simulink model "test"  (R2020a)
settings: Solver=FixedStepDiscrete  StartTime=0.0  StopTime=10.0  RelTol=1e-3
settings Model: Creator=김진성  LastModifiedBy=김진성
settings OptimizationCC: EnhancedBackFolding=on  PassReuseOutputArgsAs=Individual arguments  OptimizeBlockOrder=speed  DifferentSizesBufferReuse=on  OptimizationCustomize=off  EfficientTunableParamExpr=on
settings DebuggingCC: ParameterTunabilityLossMsg=error
settings HardwareCC: ProdBitPerPointer=32  ProdBitPerSizeT=32  ProdBitPerPtrDiffT=32  ProdLargestAtomicInteger=Long  ProdLargestAtomicFloat=Double  ProdWordSize=32  ProdHWDeviceType=ARM Compatible->ARM Cortex
settings SFSimCC: MATLABDynamicMemAlloc=off
settings RTWCC: SystemTargetFile=ert.tlc  GenCodeOnly=on  TemplateMakefile=ert_default_tmf  GenerateReport=on  IncludeHyperlinkInReport=on  LaunchReport=on  GenerateTraceInfo=on  GenerateTraceReport=on  GenerateTraceReportSl=on  GenerateTraceReportSf=on  GenerateTraceReportEml=on  GenerateCodeMetricsReport=on  GenerateCodeReplacementReport=on
settings CodeAppCC: ForceParamTrailComments=on  IgnoreCustomStorageClasses=off  OperatorAnnotations=on  SimulinkDataObjDesc=on  SFDataObjDesc=on  InsertBlockDesc=on
settings ERTTargetCC: TargetLangStandard=C99 (ISO)  GenerateSampleERTMain=on  MultiInstanceERTCode=on  CodeInterfacePackaging=Reusable function  ERTCustomFileTemplate=example_file_process.tlc

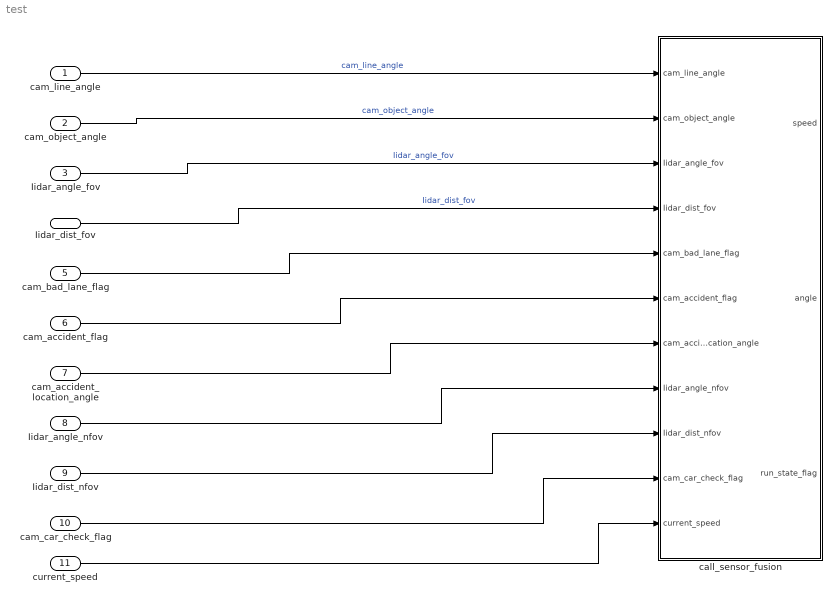
== system test ==
  cam_line_angle : Inport
  cam_object_angle : Inport  Port=2
  Iidar_angle_fov : Inport  Port=3
  Iidar_dist_fov : Inport  Port=4
  cam_bad_lane_flag : Inport  Port=5
  cam_accident_flag : Inport  Port=6
  cam_accident_location_angle : Inport  Port=7
  Iidar_angle_nfov : Inport  Port=8
  Iidar_dist_nfov : Inport  Port=9
  cam_car_check_flag : Inport  Port=10
  current_speed : Inport  Port=11
  call_sensor_fusion : Subsystem  TreatAsAtomicUnit=on
      settings: RTWSystemCode=Nonreusable function  RTWFcnNameOpts=Use subsystem name
  wires:
  cam_accident_location_angle/1 -> call_sensor_fusion/7(cam_accident_location_angle)
  cam_line_angle/1 -> call_sensor_fusion/1(cam_line_angle)  "cam_line_angle"
  cam_object_angle/1 -> call_sensor_fusion/2(cam_object_angle)  "cam_object_angle"
  Iidar_angle_fov/1 -> call_sensor_fusion/3(Iidar_angle_fov)  "Iidar_angle_fov"
  Iidar_dist_fov/1 -> call_sensor_fusion/4(Iidar_dist_fov)  "Iidar_dist_fov"
  Iidar_angle_nfov/1 -> call_sensor_fusion/8(Iidar_angle_nfov)
  Iidar_dist_nfov/1 -> call_sensor_fusion/9(Iidar_dist_nfov)
  cam_bad_lane_flag/1 -> call_sensor_fusion/5(cam_bad_lane_flag)
  cam_accident_flag/1 -> call_sensor_fusion/6(cam_accident_flag)
  cam_car_check_flag/1 -> call_sensor_fusion/10(cam_car_check_flag)
  current_speed/1 -> call_sensor_fusion/11(current_speed)

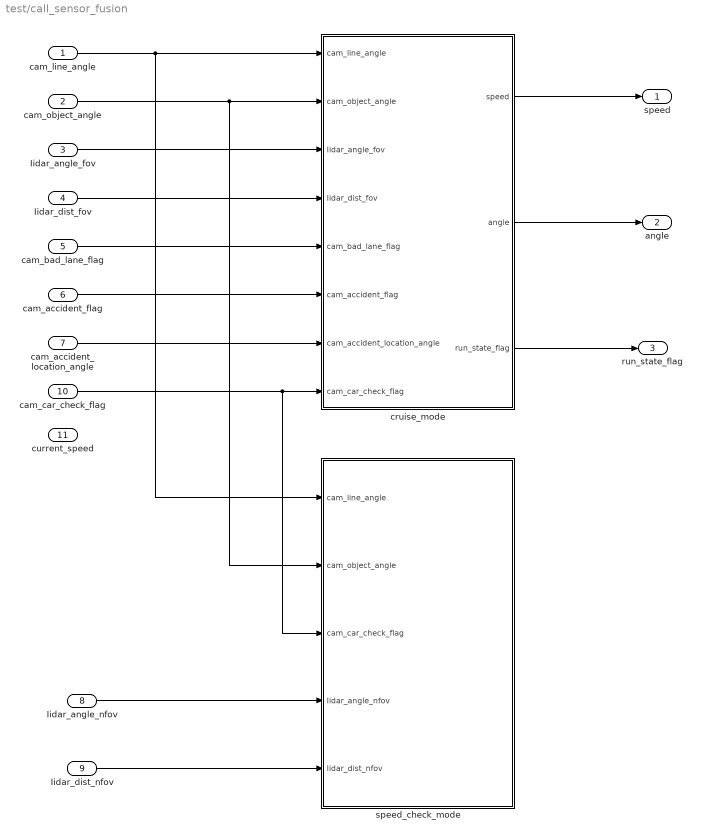
== system test/call_sensor_fusion ==
  cam_line_angle : Inport
  cam_object_angle : Inport  Port=2
  Iidar_angle_fov : Inport  Port=3
  Iidar_dist_fov : Inport  Port=4
  cam_bad_lane_flag : Inport  Port=5
  cam_accident_flag : Inport  Port=6
  cam_accident_location_angle : Inport  Port=7
  Iidar_angle_nfov : Inport  Port=8
  Iidar_dist_nfov : Inport  Port=9
  cam_car_check_flag : Inport  Port=10
  current_speed : Inport  Port=11
  cruise_mode : Subsystem  TreatAsAtomicUnit=on
      settings: RTWFcnNameOpts=Use subsystem name
  speed_check_mode : Subsystem
  speed : Outport
  angle : Outport  Port=2
  run_state_flag : Outport  Port=3
  wires:
  Iidar_angle_fov/1 -> cruise_mode/3(Iidar_angle_fov)
  Iidar_dist_fov/1 -> cruise_mode/4(Iidar_dist_fov)
  Iidar_angle_nfov/1 -> speed_check_mode/4(Iidar_angle_nfov)
  Iidar_dist_nfov/1 -> speed_check_mode/5(Iidar_dist_nfov)
  cruise_mode/2(angle) -> angle/1
  cruise_mode/1(speed) -> speed/1
  cruise_mode/3(run_state_flag) -> run_state_flag/1
  cam_line_angle/1 -> speed_check_mode/1(cam_line_angle), cruise_mode/1(cam_line_angle)
  cam_object_angle/1 -> speed_check_mode/2(cam_object_angle), cruise_mode/2(cam_object_angle)
  cam_bad_lane_flag/1 -> cruise_mode/5(cam_bad_lane_flag)
  cam_accident_flag/1 -> cruise_mode/6(cam_accident_flag)
  cam_accident_location_angle/1 -> cruise_mode/7(cam_accident_location_angle)
  cam_car_check_flag/1 -> speed_check_mode/3(cam_car_check_flag), cruise_mode/8(cam_car_check_flag)

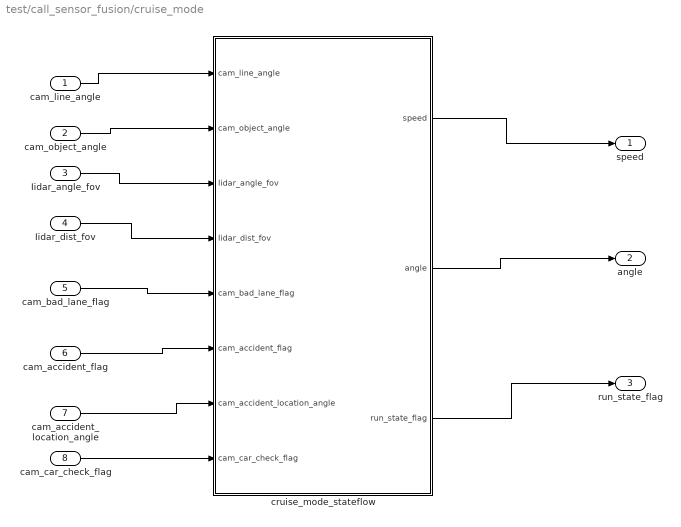
== system test/call_sensor_fusion/cruise_mode ==
  cam_line_angle : Inport
  cam_object_angle : Inport  Port=2
  Iidar_angle_fov : Inport  Port=3
  Iidar_dist_fov : Inport  Port=4
  cam_bad_lane_flag : Inport  Port=5
  cam_accident_flag : Inport  Port=6
  cam_accident_location_angle : Inport  Port=7
  cam_car_check_flag : Inport  Port=8
  cruise_mode_stateflow : Stateflow chart  TreatAsAtomicUnit=on
      settings: RTWSystemCode=Nonreusable function  RTWFcnNameOpts=Use subsystem name
  speed : Outport
  angle : Outport  Port=2
  run_state_flag : Outport  Port=3
  wires:
  cam_line_angle/1 -> cruise_mode_stateflow/1(cam_line_angle)
  cam_object_angle/1 -> cruise_mode_stateflow/2(cam_object_angle)
  cruise_mode_stateflow/1(speed) -> speed/1
  cruise_mode_stateflow/2(angle) -> angle/1
  Iidar_angle_fov/1 -> cruise_mode_stateflow/3(Iidar_angle_fov)
  Iidar_dist_fov/1 -> cruise_mode_stateflow/4(Iidar_dist_fov)
  cruise_mode_stateflow/3(run_state_flag) -> run_state_flag/1
  cam_bad_lane_flag/1 -> cruise_mode_stateflow/5(cam_bad_lane_flag)
  cam_accident_flag/1 -> cruise_mode_stateflow/6(cam_accident_flag)
  cam_accident_location_angle/1 -> cruise_mode_stateflow/7(cam_accident_location_angle)
  cam_car_check_flag/1 -> cruise_mode_stateflow/8(cam_car_check_flag)

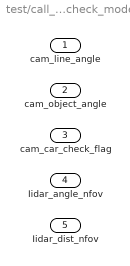
== system test/call_sensor_fusion/speed_check_mode ==
  cam_line_angle : Inport
  cam_object_angle : Inport  Port=2
  cam_car_check_flag : Inport  Port=3
  Iidar_angle_nfov : Inport  Port=4
  Iidar_dist_nfov : Inport  Port=5

== stateflow chart test/call_sensor_fusion/cruise_mode/cruise_mode_stateflow ==
  note: camera input data : cam_line_angle,
      | cam_object_angle,
      | cam_bad_lane_flag.
      | cam_accident_flag,
      | cam_accident_location_angle
  note: lidar input data : lidar_angle_fov,
      | lidar_dist_fov
  note: output data : speed,
      | angle,
      | run_state_flag
  note: 메세지 출력 -> disp("content");
  state normal_run
    % normal line following mode
    //entry:
    //local_speed = 0;
    //local_angle = 0;
    //during:
    state init
      entry:
      local_speed = 0;
      local_angle = 0;
    state routine
      entry:
    state exit
      entry:
    (default) -> init
    init -> routine
    routine -> init [order 2]
    routine -> exit [order 1]
    exit -> routine
  state calculation_front_car_speed
    % calculation of front car speed
    entry:
    exit:
  state detection_bad_lane
    % detection bad lane state
    entry:
    exit:
  state accident_occurrence
    % if accident occur
    entry:
    exit:
  (default) -> normal_run
  normal_run -> calculation_front_car_speed [order 1] : [cam_car_check_flag == 1]
  normal_run -> detection_bad_lane [order 2] : [cam_bad_lane_flag]
  normal_run -> accident_occurrence [order 3] : [cam_accident_flag]
  data: cam_line_angle input; cam_object_angle input; Iidar_angle_fov input; Iidar_dist_fov input; speed output; angle output; local_data local double; run_state_flag output double; cam_bad_lane_flag input; cam_accident_flag input; cam_accident_location_angle input; local_speed local double =0; local_angle local double =0; cam_car_check_flag input
